simulink model "power_PSS_modif"  (R2021b)
settings: Solver=ode23tb  StartTime=0.0  StopTime=20  MaxStep=1/60  RelTol=1e-3  EnableMultiTasking=on
undefined symbols (not defined in the file or in its folder): D1, Delta, M1
libraries: spsGenericPowerSystemStabilizerLib x8, spsLoadFlowBusLib x6, spsThreePhaseParallelRLCLoadLib x4, spsThreePhasePISectionLineLib x4, spsSynchronousMachinepuStandardLib x4, cstblocks x4, spsExcitationSystemLib x4, spsMultiBandPowerSystemStabilizerLib x4, spsSteamTurbineandGovernorLib x4, spsThreePhaseTransformerTwoWindingsLib x4, spsDistributedParametersLineLib x3, spsThreePhaseBreakerLib x2
(part 2 of 2)

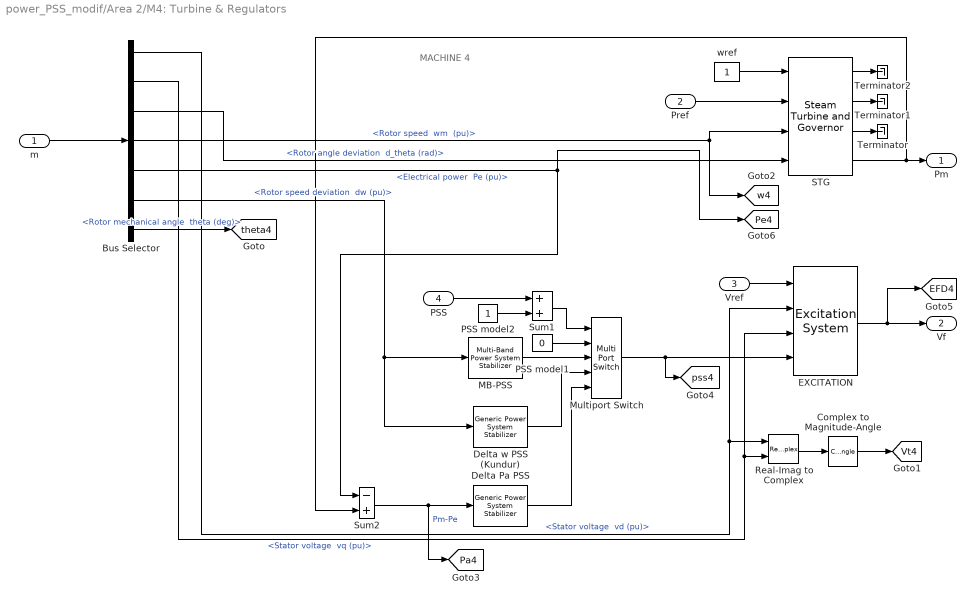
== system power_PSS_modif/Area 2/M4: Turbine & Regulators ==
  note: MACHINE 4
  m : Inport
  Pref : Inport  Port=2
  Vref : Inport  Port=3
  PSS : Inport  Port=4
  Bus Selector : BusSelector  OutputSignals="dq0 components.Stator voltage  vd (pu),dq0 components.Stator voltage  vq (pu),Mechanical.Rotor angle deviation  d_theta (rad),Mechanical.Rotor speed  wm  (pu),Mechanical.Electrical power  Pe (pu),Mechanical.Rotor speed deviation  dw (pu),Mechanical.Rotor mechanical angle  theta (deg)"
  Complex to Magnitude-Angle : ComplexToMagnitudeAngle  Output=Magnitude
  "Delta Pa PSS " : spsGenericPowerSystemStabilizerLib/Generic Power System Stabilizer  Tsensor=15e-3  K=2.5*1.25  Twashout=1  Tleadlag1=[60e-3 1]  Tleadlag2=[0 0]  VSlimits=[-0.15 0.15]  Vinit=0  Plot_On=off  MagdB_On=on  FreqRange=logspace(-2,2,500)
      settings: SourceProductBaseCode=PS
  "Delta w PSS (Kundur) " : spsGenericPowerSystemStabilizerLib/Generic Power System Stabilizer  Tsensor=15e-3  K=30  Twashout=10  Tleadlag1=[50e-3 20e-3]  Tleadlag2=[3 5.4]  VSlimits=[-0.15 0.15]  Vinit=0  Plot_On=off  MagdB_On=on  FreqRange=logspace(-2,2,500)
      settings: SourceProductBaseCode=PS
  EXCITATION : spsExcitationSystemLib/Excitation System  tr=20e-3  reg=[ 200, 0.001 ]  exc=[ 1, 0 ]  tgr=[ 0, 0 ]  damp=[ 0, 0 ]  sat=[ 0, 0 ]  lim=[ 0 , 12.3, 0 ]  v0=[1,1.82209]
      settings: SourceProductBaseCode=PS
  "MB-PSS " : spsMultiBandPowerSystemStabilizerLib/Multi-Band Power System Stabilizer  OperationMode=Simplified settings  Kg=1.0  GL=[0.2 30]  GI=[1.25 40]  GH=[12.0 160]  GLd=[66 66 9.4]  TcLF=[1.667 2 0 0 0 0 2 2.4 0 0 0 0 1 1]  GId=[66 66 47.6]  TcIF=[1 1 0.25 0.3 0 0 1 1 0.3 0.36 0 0 0 0]  GHd=[66 66 233]  TcHF="[0.01 0.012 0 0 0 0  0.012 0.0144 0 0 0 0 1 1]"  LIM=[.075 .15 .15 .15]  Plot_On=off  MagdB_On=off  FreqRange=logspace(-2,2,500)
      settings: SourceProductBaseCode=PS
  Multiport Switch : MultiPortSwitch  Inputs=4  InputSameDT=on
  PSS model1 : Constant  Value=0
  PSS model2 : Constant
  Real-Imag to Complex : RealImagToComplex
  STG : spsSteamTurbineandGovernorLib/Steam Turbine and Governor  gentype=Tandem-compound (single mass)  reg1="[ 1  0.05    0 ]"  reg2="[ 0.001  0.15 ]"  reg3="[ -0.1  0.1  0  4.496 ]"  N=3600  turb1="[ 0  10   3.3   0.5   ]"  turb2="[   0   0.36    0.36   0.28   ]"  HA="[ 0.046  1.430  1.465   0.192 ]"  KA="[ 90.44  53.88  64.59   62.94  ]"  DA="[ 0.0115  0.3575  0.3663   0.0137  ]"  ini1=0.7778  ini2=[0.779311,-67.7513]
      settings: SourceProductBaseCode=PS
  Sum1 : Sum  InputSameDT=on  SaturateOnIntegerOverflow=on  OutDataTypeStr=Inherit: Same as first input
  Sum2 : Sum  Inputs=-+  InputSameDT=on  SaturateOnIntegerOverflow=on  OutDataTypeStr=Inherit: Same as first input
  Terminator : Terminator
  Terminator1 : Terminator
  Terminator2 : Terminator
  wref : Constant
  Pm : Outport  InitialOutput=0  VectorParamsAs1DForOutWhenUnconnected=off
  Vf : Outport  Port=2  InitialOutput=0  VectorParamsAs1DForOutWhenUnconnected=off
  tag scope: EFD4=global, Pa4=global, Pe4=global, Vt4=global, pss4=global, theta4=global, w4=global
  wires:
  Bus Selector/1 -> EXCITATION/2, Real-Imag to Complex/1  "<Stator voltage  vd (pu)>"
  Bus Selector/2 -> EXCITATION/3, Real-Imag to Complex/2  "<Stator voltage  vq (pu)>"
  STG/4 -> Pm/1, Sum2/2
  wref/1 -> STG/1
  Pref/1 -> STG/2
  Vref/1 -> EXCITATION/1
  STG/3 -> Terminator/1
  Real-Imag to Complex/1 -> Complex to Magnitude-Angle/1
  EXCITATION/1 -> Vf/1, [EFD4]
  Complex to Magnitude-Angle/1 -> [Vt4]
  Bus Selector/7 -> [theta4]  "<Rotor mechanical angle  theta (deg)>"
  Multiport Switch/1 -> EXCITATION/4, [pss4]
  PSS model1/1 -> Multiport Switch/2
  "MB-PSS "/1 -> Multiport Switch/3
  "Delta w PSS (Kundur) "/1 -> Multiport Switch/4
  "Delta Pa PSS "/1 -> Multiport Switch/5
  PSS model2/1 -> Sum1/2
  Sum1/1 -> Multiport Switch/1
  PSS/1 -> Sum1/1
  Bus Selector/4 -> STG/3, [w4]  "<Rotor speed  wm  (pu)>"
  Bus Selector/5 -> [Pe4], Sum2/1  "<Electrical power  Pe (pu)>"
  Bus Selector/6 -> "MB-PSS "/1, "Delta w PSS (Kundur) "/1  "<Rotor speed deviation  dw (pu)>"
  Sum2/1 -> [Pa4], "Delta Pa PSS "/1  "Pm-Pe"
  STG/2 -> Terminator1/1
  STG/1 -> Terminator2/1
  Bus Selector/3 -> STG/4  "<Rotor angle deviation  d_theta (rad)>"
  m/1 -> Bus Selector/1

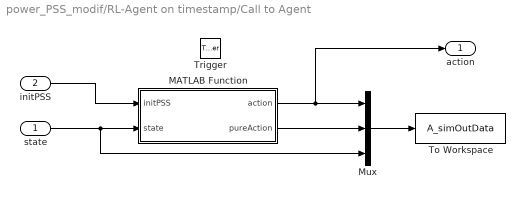
== system power_PSS_modif/RL-Agent on timestamp/Call to Agent ==
  state : Inport
  initPSS : Inport  Port=2
  Trigger : TriggerPort  VariantControl=(inherit)  InitialTriggerSignalState=positive  PortDimensions=1
  MATLAB Function : MATLAB Function  TreatAsAtomicUnit=on
  Mux : Mux  Inputs=3
  To Workspace : ToWorkspace  VariableName=A_simOutData  SampleTime=-1
  action : Outport
  wires:
  Mux/1 -> To Workspace/1
  state/1 -> Mux/3, MATLAB Function/2(state)
  MATLAB Function/2(pureAction) -> Mux/2
  MATLAB Function/1(action) -> action/1, Mux/1
  initPSS/1 -> MATLAB Function/1(initPSS)

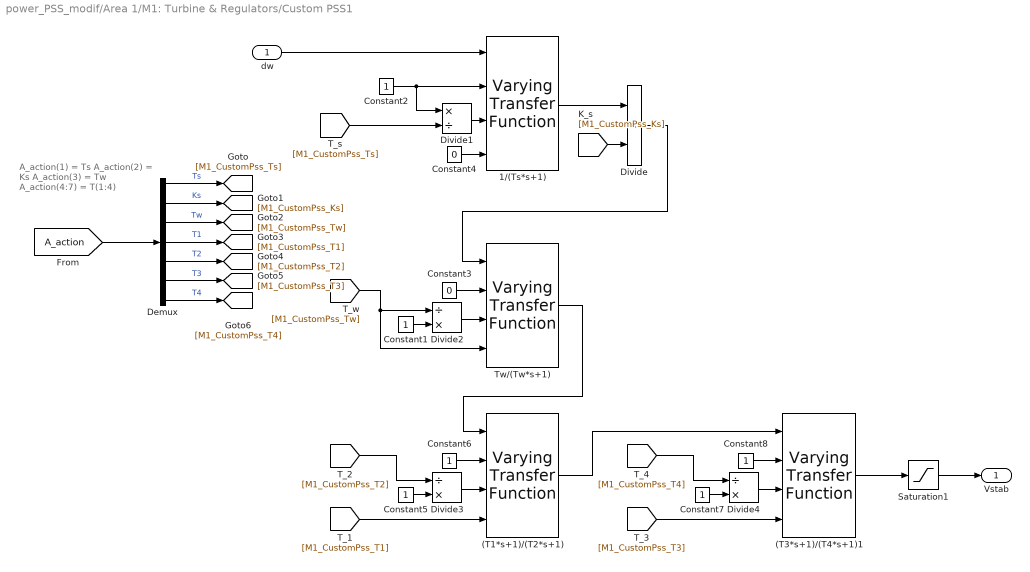
== system power_PSS_modif/Area 1/M1: Turbine & Regulators/Custom PSS1 ==
  note: A_action(1) = Ts
      | A_action(2) = Ks
      | A_action(3) = Tw
      | A_action(4:7) = T(1:4)
  dw : Inport
  (T1*s+1)/(T2*s+1) : cstblocks/Linear Parameter Varying/Varying Transfer Function  N=1
  (T3*s+1)/(T4*s+1)1 : cstblocks/Linear Parameter Varying/Varying Transfer Function  N=1
  1/(Ts*s+1) : cstblocks/Linear Parameter Varying/Varying Transfer Function  N=1
  Constant{1..2,5..8} (6 alike) : Constant
  Constant3 : Constant  Value=0
  Constant4 : Constant  Value=0
  Demux : Demux  Outputs=7
  Divide : Product  Inputs=**
  Divide1 : Product  Inputs=*/
  Divide2 : Product  Inputs=/*
  Divide3 : Product  Inputs=/*
  Divide4 : Product  Inputs=/*
  Saturation1 : Saturate  UpperLimit=M1.CustomPSS1.Upper  LowerLimit=M1.CustomPSS1.Lower
  Tw/(Tw*s+1) : cstblocks/Linear Parameter Varying/Varying Transfer Function  N=1
  Vstab : Outport
  wires:
  dw/1 -> 1/(Ts*s+1)/1
  1/(Ts*s+1)/1 -> Divide/1
  Divide/1 -> Tw/(Tw*s+1)/1
  Demux/1 -> [M1_CustomPss_Ts]  "Ts"
  Demux/2 -> [M1_CustomPss_Ks]  "Ks"
  Demux/3 -> [M1_CustomPss_Tw]  "Tw"
  Demux/4 -> [M1_CustomPss_T1]  "T1"
  Demux/5 -> [M1_CustomPss_T2]  "T2"
  Demux/6 -> [M1_CustomPss_T3]  "T3"
  Demux/7 -> [M1_CustomPss_T4]  "T4"
  [M1_CustomPss_Ks] -> Divide/2
  Divide1/1 -> 1/(Ts*s+1)/3
  Constant2/1 -> 1/(Ts*s+1)/2, Divide1/1
  Constant4/1 -> 1/(Ts*s+1)/4
  [M1_CustomPss_Tw] -> Divide2/1, Tw/(Tw*s+1)/4
  Constant1/1 -> Divide2/2
  Divide2/1 -> Tw/(Tw*s+1)/3
  Saturation1/1 -> Vstab/1
  Tw/(Tw*s+1)/1 -> (T1*s+1)/(T2*s+1)/1
  Constant3/1 -> Tw/(Tw*s+1)/2
  Divide3/1 -> (T1*s+1)/(T2*s+1)/3
  Constant6/1 -> (T1*s+1)/(T2*s+1)/2
  [M1_CustomPss_T2] -> Divide3/1
  Constant5/1 -> Divide3/2
  [M1_CustomPss_T1] -> (T1*s+1)/(T2*s+1)/4
  [M1_CustomPss_T4] -> Divide4/1
  Constant8/1 -> (T3*s+1)/(T4*s+1)1/2
  Divide4/1 -> (T3*s+1)/(T4*s+1)1/3
  Constant7/1 -> Divide4/2
  [M1_CustomPss_T3] -> (T3*s+1)/(T4*s+1)1/4
  (T1*s+1)/(T2*s+1)/1 -> (T3*s+1)/(T4*s+1)1/1
  (T3*s+1)/(T4*s+1)1/1 -> Saturation1/1
  [M1_CustomPss_Ts] -> Divide1/2
  [A_action] -> Demux/1

== matlab function power_PSS_modif/RL-Agent on timestamp/MATLAB Function ==
  data: time input; isTime output; period input
function isTime = trigger(time, period)
    if (mod(time, period))
        isTime = 0;
        return;
    end
    isTime = 1;
end

== matlab function power_PSS_modif/RL-Agent on timestamp/Call to Agent/MATLAB Function ==
  data: initPSS input; state input; action output; pureAction output
function [action, pureAction] = agent(initPSS, state)
    % Инициализация, требуемая компилятором
    % Размерность зависит от того, на какой тип регулятора подается
    % воздействие агента.
    %
    % NOTE: Привязать размерность к типу регулятора и вынести на верхний
    % уровень модели
    action = initPSS;
    pureAction = initPSS;

    % Вызов внешней m-функции-обёртки над pyrunfile.
    % Инспирированно несовместимой реализацией компилятора Simulink.
    % Внутри блока MATLAB Function множество синтаксических возможностей,
    % которые доступны в матлабе, не реализованы и просто не обрабатываются
    % парсером. Для рассматриваемой задачи это критично ввиду того, что
    % внутри этого блока не получится скастить py.list, получаемый из
    % py-функции, к требуемому типу mxArray, а в следствии и к double.
    coder.extrinsic('matAgentCall');
    [action, pureAction] = matAgentCall(state);
end

== matlab function power_PSS_modif/RL-Agent on timestamp/MATLAB Function1 ==
  data: time input; period input; outData output; data input; initPSS input
function outData = delay(time, period, data, initPSS)
    outData = initPSS;
    
    coder.extrinsic('actionDelay');
    outData = actionDelay(time, period, data, initPSS);
end
